simulink model "model_sim_CHBjt5"  (R2023b)
settings: Solver=FixedStepAuto  StartTime=0.0  StopTime=5  FixedStep=1e-6  RelTol=1e-3
InitFcn:
  | sysinit
StopFcn:
  | code_CHBJT5_stopfcn
values from neighbouring files (symbols this model uses):
  C = 0.0234    [sysinit.m]
  f = 50    [sysinit.m]
  f_switch = 250    [sysinit.m]
  fn = 50    [sysinit.m]
  L = 0.002    [sysinit.m]
  L_ori = 0.02    [sysinit.m]
  L_sec = 0.06    [sysinit.m]
  m = 0.95    [sysinit.m]
  P0 = 8e6    (= 8000000)    [sysinit.m]
  R = 1.5    [sysinit.m]
  Source_Amp = 10000    [sysinit.m]
  st = 1e-6    (= 1e-06)    [sysinit.m]
  Td = 15e-7    (= 1.5e-06)    [sysinit.m]
  Ts2 = 0.5e-3    (= 0.0005)    [sysinit.m]
  U_dcN = 2500    [sysinit.m]
  Ul_in = 1900    [sysinit.m]
undefined symbols (not defined in the file or in its folder): D1, Delta, magnitude
libraries: spsSeriesRLCBranchLib x63, spsDiodeLib x30, simulink x26, spsIGBTLib x24, spsMeanLib x20, spsCurrentMeasurementLib x10, spsThreePhaseVIMeasurementLib x7, spsOnDelayLib x6, spsUniversalBridgeLib x6, spsRMSLib x4, spsVoltageMeasurementLib x3, spsThreePhaseTransformerThreeWindingsLib x3
(part 1 of 2)
settings Model: SimulationMode=accelerator  Creator=Jhchen  LastModifiedBy=Jhchen
settings DataIOCC: ReturnWorkspaceOutputs=off
settings DebuggingCC: RTPrefix=warning

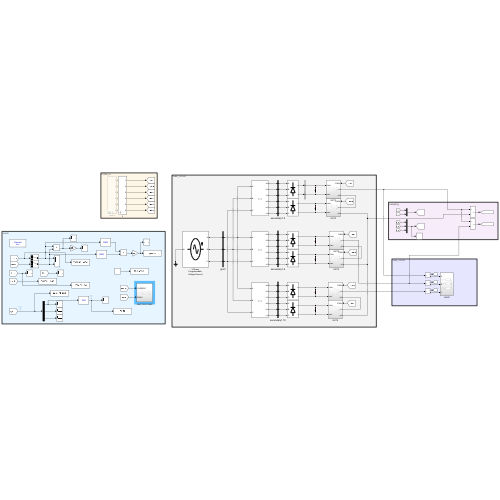
[thumbnail: Simulink's stored preview of the top-level diagram]
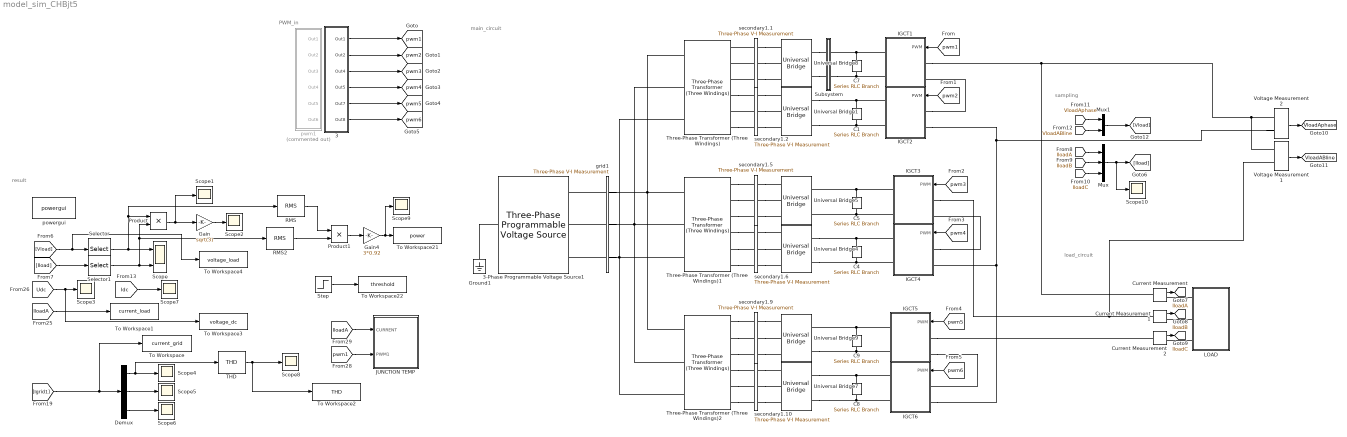
== system model_sim_CHBjt5 ==
  note: load_circuit
  note: main_circuit
  note: PWM_in
  note: result
  note: sampling
  3 : Subsystem  mask{m=m, f=f, f_car=f_switch, tt=1/4, ttd=Td}
      mask prompts: m "m_p"; f "f_module"; f_car "f_carrier"; tt "ts"; ttd "td"
      mask DialogControl ParameterGroupVar Prompt: 参数
  3-Phase Programmable Voltage Source1 : spsThreePhaseProgrammableVoltageSourceLib/Three-Phase Programmable Voltage Source  PositiveSequence=[10000 0 50]  VariationEntity=None  VariationType=Step  VariationTypeAlt=Step  VariationStep=0.5  VariationRate=10  VariationMagnitude=0.3  VariationFrequency=2  VariationTiming=[0.05 1]  VariationPhaseA=off  Amplitudes=[1 0.8 1.2 1.0]  TimeValues=[0 0.1 0.15 0.2]  HarmonicGeneration=off  HarmonicA=[5 0.08 -45 2]  HarmonicB=[2 0 0 2]  Timing="[0.1  1]"  BusType=swing  Pref=0  Qref=0  Qmin=-inf  Qmax=inf
  C{1,4..5,7..9} (6 alike) : spsSeriesRLCBranchLib/Series RLC Branch  LConnTagsString=__new0  RConnTagsString=__new0  BranchType=C  Resistance=0.0001  Inductance=1.0  SetiL0=off  InitialCurrent=0  Capacitance=C  Setx0=on  InitialVoltage=2500  Measurements=None
  Current Measurement : spsCurrentMeasurementLib/Current Measurement  PhasorSimulation=off  OutputType=Complex  PSBequivalent=0
  Current Measurement1 : spsCurrentMeasurementLib/Current Measurement  PhasorSimulation=off  OutputType=Complex  PSBequivalent=0
  Current Measurement2 : spsCurrentMeasurementLib/Current Measurement  PhasorSimulation=off  OutputType=Complex  PSBequivalent=0
  Demux : Demux  Outputs=3
  Gain : Gain  Gain=sqrt(3)
  Gain4 : Gain  Gain=3*0.92
  Ground1 : spsGroundLib/Ground  LConnTagsString=a
  IGCT1 : Subsystem
      settings: PortSchema="{\"entries\":[{\"content\":{\"sides\":[{\"content\":{\"connectorIds\":[\"LConn1\",\"LConn2\"]},\"type\":\"ConnectorPlacement.EquallySpacedRectSide\",\"uuid\":\"3b5227fd-32cc-4097-9a6a-2909540651e9\"},{\"content\":{\"connectorIds\":[\"In1\",\"RConn1\",\"RConn2\"],\"side\":\"RIGHT\"},\"type\":\"ConnectorPlacement.EquallySpacedRectSide\",\"uuid\":\"b0068562-9d9a-456b-acd2-db870c5bcace\"},{\"content\":{\"side\":\"TOP\"},\"type\":\"ConnectorPlacement.EquallySpacedRectSide\",\"uuid\":\"bbecbe08-a8e7-4703-9f6f-443f87d924da\"}]},\"type\":\"ConnectorPlacement.EquallySpacedConnector\",\"uuid\":\"6ec83c7b-e3bb-4502-bc8f-4da9ff103a20\"}],\"packageUris\":[\"http://schema.mathworks.com/mf0/Connector/R2020b\"],\"version\":\"1.0\"}"
  IGCT2 : Subsystem
      settings: PortSchema="{\"entries\":[{\"content\":{\"sides\":[{\"content\":{\"connectorIds\":[\"LConn1\",\"LConn2\"]},\"type\":\"ConnectorPlacement.EquallySpacedRectSide\",\"uuid\":\"3b5227fd-32cc-4097-9a6a-2909540651e9\"},{\"content\":{\"connectorIds\":[\"In1\",\"RConn1\",\"RConn2\"],\"side\":\"RIGHT\"},\"type\":\"ConnectorPlacement.EquallySpacedRectSide\",\"uuid\":\"b0068562-9d9a-456b-acd2-db870c5bcace\"},{\"content\":{\"side\":\"TOP\"},\"type\":\"ConnectorPlacement.EquallySpacedRectSide\",\"uuid\":\"bbecbe08-a8e7-4703-9f6f-443f87d924da\"}]},\"type\":\"ConnectorPlacement.EquallySpacedConnector\",\"uuid\":\"6ec83c7b-e3bb-4502-bc8f-4da9ff103a20\"}],\"packageUris\":[\"http://schema.mathworks.com/mf0/Connector/R2020b\"],\"version\":\"1.0\"}"
  IGCT3 : Subsystem
      settings: PortSchema="{\"entries\":[{\"content\":{\"sides\":[{\"content\":{\"connectorIds\":[\"LConn1\",\"LConn2\"]},\"type\":\"ConnectorPlacement.EquallySpacedRectSide\",\"uuid\":\"3b5227fd-32cc-4097-9a6a-2909540651e9\"},{\"content\":{\"connectorIds\":[\"In1\",\"RConn1\",\"RConn2\"],\"side\":\"RIGHT\"},\"type\":\"ConnectorPlacement.EquallySpacedRectSide\",\"uuid\":\"b0068562-9d9a-456b-acd2-db870c5bcace\"},{\"content\":{\"side\":\"TOP\"},\"type\":\"ConnectorPlacement.EquallySpacedRectSide\",\"uuid\":\"bbecbe08-a8e7-4703-9f6f-443f87d924da\"}]},\"type\":\"ConnectorPlacement.EquallySpacedConnector\",\"uuid\":\"6ec83c7b-e3bb-4502-bc8f-4da9ff103a20\"}],\"packageUris\":[\"http://schema.mathworks.com/mf0/Connector/R2020b\"],\"version\":\"1.0\"}"
  IGCT4 : Subsystem
      settings: PortSchema="{\"entries\":[{\"content\":{\"sides\":[{\"content\":{\"connectorIds\":[\"LConn1\",\"LConn2\"]},\"type\":\"ConnectorPlacement.EquallySpacedRectSide\",\"uuid\":\"3b5227fd-32cc-4097-9a6a-2909540651e9\"},{\"content\":{\"connectorIds\":[\"In1\",\"RConn1\",\"RConn2\"],\"side\":\"RIGHT\"},\"type\":\"ConnectorPlacement.EquallySpacedRectSide\",\"uuid\":\"b0068562-9d9a-456b-acd2-db870c5bcace\"},{\"content\":{\"side\":\"TOP\"},\"type\":\"ConnectorPlacement.EquallySpacedRectSide\",\"uuid\":\"bbecbe08-a8e7-4703-9f6f-443f87d924da\"}]},\"type\":\"ConnectorPlacement.EquallySpacedConnector\",\"uuid\":\"6ec83c7b-e3bb-4502-bc8f-4da9ff103a20\"}],\"packageUris\":[\"http://schema.mathworks.com/mf0/Connector/R2020b\"],\"version\":\"1.0\"}"
  IGCT5 : Subsystem
      settings: PortSchema="{\"entries\":[{\"content\":{\"sides\":[{\"content\":{\"connectorIds\":[\"LConn1\",\"LConn2\"]},\"type\":\"ConnectorPlacement.EquallySpacedRectSide\",\"uuid\":\"3b5227fd-32cc-4097-9a6a-2909540651e9\"},{\"content\":{\"connectorIds\":[\"In1\",\"RConn1\",\"RConn2\"],\"side\":\"RIGHT\"},\"type\":\"ConnectorPlacement.EquallySpacedRectSide\",\"uuid\":\"b0068562-9d9a-456b-acd2-db870c5bcace\"},{\"content\":{\"side\":\"TOP\"},\"type\":\"ConnectorPlacement.EquallySpacedRectSide\",\"uuid\":\"bbecbe08-a8e7-4703-9f6f-443f87d924da\"}]},\"type\":\"ConnectorPlacement.EquallySpacedConnector\",\"uuid\":\"6ec83c7b-e3bb-4502-bc8f-4da9ff103a20\"}],\"packageUris\":[\"http://schema.mathworks.com/mf0/Connector/R2020b\"],\"version\":\"1.0\"}"
  IGCT6 : Subsystem
      settings: PortSchema="{\"entries\":[{\"content\":{\"sides\":[{\"content\":{\"connectorIds\":[\"LConn1\",\"LConn2\"]},\"type\":\"ConnectorPlacement.EquallySpacedRectSide\",\"uuid\":\"3b5227fd-32cc-4097-9a6a-2909540651e9\"},{\"content\":{\"connectorIds\":[\"In1\",\"RConn1\",\"RConn2\"],\"side\":\"RIGHT\"},\"type\":\"ConnectorPlacement.EquallySpacedRectSide\",\"uuid\":\"b0068562-9d9a-456b-acd2-db870c5bcace\"},{\"content\":{\"side\":\"TOP\"},\"type\":\"ConnectorPlacement.EquallySpacedRectSide\",\"uuid\":\"bbecbe08-a8e7-4703-9f6f-443f87d924da\"}]},\"type\":\"ConnectorPlacement.EquallySpacedConnector\",\"uuid\":\"6ec83c7b-e3bb-4502-bc8f-4da9ff103a20\"}],\"packageUris\":[\"http://schema.mathworks.com/mf0/Connector/R2020b\"],\"version\":\"1.0\"}"
  JUNCTION TEMP : Subsystem
  LOAD : Subsystem
  Mux : Mux  Inputs=3
  Mux1 : Mux  Inputs=2
  Product : Product
  Product1 : Product
  RMS : spsRMSLib/RMS  TrueRMS=on  Freq=f  RMSInit=0  Ts=0
  RMS2 : spsRMSLib/RMS  TrueRMS=on  Freq=f  RMSInit=0  Ts=0
  Scope : Scope  NumInputPorts=2
  Scope{1..10} (10 alike) : Scope
  Selector : Selector  InputPortWidth=2  IndexOptions=Index vector (dialog)  Indices=[1]  OutputSizes=1
  Selector1 : Selector  InputPortWidth=3  IndexOptions=Index vector (dialog)  Indices=[1]  OutputSizes=1
  Step : Step  Time=0  Before=140  After=140  SampleTime=0
  Subsystem : Subsystem
  THD : spsTHDLib/THD  Freq=f  Ts=0
  Three-Phase Transformer (Three Windings) : spsThreePhaseTransformerThreeWindingsLib/Three-Phase Transformer (Three Windings)  Winding1Connection=Y  Winding2Connection=Y  Winding3Connection=Delta (D1)  CoreType=Three single-phase transformers  SetSaturation=off  Hysteresis=off  DataFile='hysteresis'  SetInitialFlux=off  Measurements=None  UNITS=pu  NominalPower=[ P0, fn ]  Winding1=[Source_Amp 0.002 L_ori]  Winding2=[Ul_in 0.002 L_sec]  Winding3=[Ul_in 0.002 L_sec]  Rm=500  Lm=499.99  L0=0.5  Saturation=[0 0;0.0024 1.2;1 1.5199]  InitialFluxes=[0.8 -0.8 0.7]  BreakLoop=off  DiscreteSolver=Trapezoidal iterative  DataType=off  TransfoNumber=1
      settings: LibrarySourceBlock=|
      | sps_lib/Power Grid Elements/Three-Phase
      | Transformer
      | (Three Windings)
  Three-Phase Transformer (Three Windings)1 : spsThreePhaseTransformerThreeWindingsLib/Three-Phase Transformer (Three Windings)  Winding1Connection=Y  Winding2Connection=Y  Winding3Connection=Delta (D1)  CoreType=Three single-phase transformers  SetSaturation=off  Hysteresis=off  DataFile='hysteresis'  SetInitialFlux=off  Measurements=None  UNITS=pu  NominalPower=[ P0, fn ]  Winding1=[Source_Amp 0.002 L_ori]  Winding2=[Ul_in 0.002 L_sec]  Winding3=[Ul_in 0.002 L_sec]  Rm=500  Lm=499.99  L0=0.5  Saturation=[0 0;0.0024 1.2;1 1.5199]  InitialFluxes=[0.8 -0.8 0.7]  BreakLoop=off  DiscreteSolver=Trapezoidal iterative  DataType=off  TransfoNumber=1
      settings: LibrarySourceBlock=|
      | sps_lib/Power Grid Elements/Three-Phase
      | Transformer
      | (Three Windings)
  Three-Phase Transformer (Three Windings)2 : spsThreePhaseTransformerThreeWindingsLib/Three-Phase Transformer (Three Windings)  Winding1Connection=Y  Winding2Connection=Y  Winding3Connection=Delta (D1)  CoreType=Three single-phase transformers  SetSaturation=off  Hysteresis=off  DataFile='hysteresis'  SetInitialFlux=off  Measurements=None  UNITS=pu  NominalPower=[ P0, fn ]  Winding1=[Source_Amp 0.002 L_ori]  Winding2=[Ul_in 0.002 L_sec]  Winding3=[Ul_in 0.002 L_sec]  Rm=500  Lm=499.99  L0=0.5  Saturation=[0 0;0.0024 1.2;1 1.5199]  InitialFluxes=[0.8 -0.8 0.7]  BreakLoop=off  DiscreteSolver=Trapezoidal iterative  DataType=off  TransfoNumber=1
      settings: LibrarySourceBlock=|
      | sps_lib/Power Grid Elements/Three-Phase
      | Transformer
      | (Three Windings)
  To Workspace : ToWorkspace  VariableName=current_grid  SaveFormat=Structure With Time  SampleTime=-1
  To Workspace1 : ToWorkspace  VariableName=current_load  SaveFormat=Structure With Time  SampleTime=-1
  To Workspace2 : ToWorkspace  VariableName=THD  SaveFormat=Structure With Time  SampleTime=-1
  To Workspace21 : ToWorkspace  VariableName=power  SaveFormat=Structure With Time  SampleTime=-1
  To Workspace22 : ToWorkspace  VariableName=threshold  SaveFormat=Structure With Time  SampleTime=-1
  To Workspace3 : ToWorkspace  VariableName=voltage_dc  SaveFormat=Structure With Time  SampleTime=-1
  To Workspace4 : ToWorkspace  VariableName=voltage_load  SaveFormat=Structure With Time  SampleTime=-1
  Universal Bridge{1,4..5,7..9} (6 alike) : spsUniversalBridgeLib/Universal Bridge  Arms=3  SnubberResistance=1e5  SnubberCapacitance=inf  Device=Diodes  Ron=1e-3  Lon=0  ForwardVoltages="[  0  0  ]"  ForwardVoltage=0  GTOparameters=[ 10e-6 , 20e-6 ]  IGBTparameters=[ 1e-6 , 2e-6 ]  Measurements=None  Measurements_2=None  converterType=Rectifier
  Voltage Measurement1 : spsVoltageMeasurementLib/Voltage Measurement  PhasorSimulation=off  OutputType=Complex  PSBequivalent=0
  Voltage Measurement2 : spsVoltageMeasurementLib/Voltage Measurement  PhasorSimulation=off  OutputType=Complex  PSBequivalent=0
  grid1 : spsThreePhaseVIMeasurementLib/Three-Phase V-I Measurement  VoltageMeasurement=phase-to-ground  SetLabelV=on  LabelV=Vgrid1  Vpu=off  VpuLL=off  CurrentMeasurement=yes  SetLabelI=on  LabelI=Igrid1  Ipu=off  Pbase=1e3  Vbase=380  OutputType=Magnitude  PhasorSimulation=off  PSBequivalent=0
  powergui : spspowerguiLib/powergui  Priority=1  SimulationMode=Discrete  SampleTime=st  frequency=60  Iterations=50  frequencyindice=50  Pbase=100e6  ErrMax=1e-4  UnitsV=kV  UnitsW=MW  buscounter=0  FunctionMessages=off  echomessages=off  EnableUseOfTLC=off  CurrentSourceSwitches=off  DisableSnubberDevices=off  DisableRonSwitches=off  DisableVfSwitches=off  DisplayEquations=off  AutomaticDiscreteSolvers=off  SolverType=Tustin/Backward Euler (TBE)  Interpol=off  ExternalGateDelay=off  methode=off  Ts=100  x0status=blocks  SPID=on  SwTol=0  HookPort=off  NonlinearTolerance=1e-4  nMaxIteration=100  ContinueOnMaxIteration=off  RestoreLinks=warning  ResistiveCurrentMeasurement=off  Frange=[0:2:500]  Ylog=off  Xlog=on  ShowGrid=off  save=off  variable=ZData  structure=0  ZoomFFT=off  StartTime=0.0  cycles=1  DisplayStyle=1  fundamental=60  FreqAxis=off  MaxFrequency=1000  frequencyindicesteady=1  RmsSteady=1  display=off
  pwm1 : Subsystem  Commented=on  mask{m=0.95, f=50, f_carrier=250, sw1=TRIBLE_SINE, sw=PS4}
      mask prompts: m "m_p"; f "f_module"; sw1 "mod"; sw "pwm_out"
      mask TypeOptions sw1: SINE | TRIBLE_SINE | GDSINE1 | GDSINE2
      mask TypeOptions sw: PS4 | POD1 | PD2
  secondary1.1 : spsThreePhaseVIMeasurementLib/Three-Phase V-I Measurement  VoltageMeasurement=phase-to-phase  SetLabelV=on  LabelV=Vsecondary_a1  Vpu=off  VpuLL=off  CurrentMeasurement=yes  SetLabelI=on  LabelI=Isecondary_a1  Ipu=off  Pbase=1e3  Vbase=380  OutputType=Magnitude  PhasorSimulation=off  PSBequivalent=0
  secondary1.10 : spsThreePhaseVIMeasurementLib/Three-Phase V-I Measurement  VoltageMeasurement=phase-to-phase  SetLabelV=on  LabelV=Vsecondary_c2  Vpu=off  VpuLL=off  CurrentMeasurement=yes  SetLabelI=on  LabelI=Isecondary_c2  Ipu=off  Pbase=1e3  Vbase=380  OutputType=Magnitude  PhasorSimulation=off  PSBequivalent=0
  secondary1.2 : spsThreePhaseVIMeasurementLib/Three-Phase V-I Measurement  VoltageMeasurement=phase-to-phase  SetLabelV=on  LabelV=Vsecondary_a2  Vpu=off  VpuLL=off  CurrentMeasurement=yes  SetLabelI=on  LabelI=Isecondary_a2  Ipu=off  Pbase=1e3  Vbase=380  OutputType=Magnitude  PhasorSimulation=off  PSBequivalent=0
  secondary1.5 : spsThreePhaseVIMeasurementLib/Three-Phase V-I Measurement  VoltageMeasurement=phase-to-phase  SetLabelV=on  LabelV=Vsecondary_b1  Vpu=off  VpuLL=off  CurrentMeasurement=yes  SetLabelI=on  LabelI=Isecondary_b1  Ipu=off  Pbase=1e3  Vbase=380  OutputType=Magnitude  PhasorSimulation=off  PSBequivalent=0
  secondary1.6 : spsThreePhaseVIMeasurementLib/Three-Phase V-I Measurement  VoltageMeasurement=phase-to-phase  SetLabelV=on  LabelV=Vsecondary_b2  Vpu=off  VpuLL=off  CurrentMeasurement=yes  SetLabelI=on  LabelI=Isecondary_b2  Ipu=off  Pbase=1e3  Vbase=380  OutputType=Magnitude  PhasorSimulation=off  PSBequivalent=0
  secondary1.9 : spsThreePhaseVIMeasurementLib/Three-Phase V-I Measurement  VoltageMeasurement=phase-to-phase  SetLabelV=on  LabelV=Vsecondary_c1  Vpu=off  VpuLL=off  CurrentMeasurement=yes  SetLabelI=on  LabelI=Isecondary_c1  Ipu=off  Pbase=1e3  Vbase=380  OutputType=Magnitude  PhasorSimulation=off  PSBequivalent=0
  tag scope: IloadA=global, IloadB=global, IloadC=global, VloadABline=global, VloadAphase=global, pwm1=global, pwm2=global, pwm3=global, pwm4=global, pwm5=global, pwm6=global
  wires:
  [pwm1] -> IGCT1/1(PWM)
  [pwm2] -> IGCT2/1(PWM)
  [pwm3] -> IGCT3/1(PWM)
  [pwm4] -> IGCT4/1(PWM)
  [pwm5] -> IGCT5/1(PWM)
  [pwm6] -> IGCT6/1(PWM)
  [Vload] -> To Workspace4/1, Selector/1
  Selector/1 -> Product/1, RMS/1, Scope/1
  [Iload] -> Selector1/1
  Selector1/1 -> Product/2, RMS2/1, Scope/2
  Current Measurement/1 -> [IloadA]
  Current Measurement1/1 -> [IloadB]
  Current Measurement2/1 -> [IloadC]
  [IloadC] -> Mux/3
  [IloadB] -> Mux/2
  [IloadA] -> Mux/1
  Mux/1 -> Scope10/1, [Iload]
  Voltage Measurement2/1 -> [VloadAphase]
  Voltage Measurement1/1 -> [VloadABline]
  [VloadAphase] -> Mux1/1
  [VloadABline] -> Mux1/2
  Mux1/1 -> [Vload]
  Product/1 -> Scope1/1, Gain/1
  Gain/1 -> Scope2/1
  [IloadA] -> To Workspace1/1
  [Udc] -> To Workspace3/1, Scope3/1
  3/1(Out1) -> [pwm1]
  3/2(Out2) -> [pwm2]
  3/3(Out4) -> [pwm3]
  3/4(Out5) -> [pwm4]
  3/5(Out7) -> [pwm5]
  3/6(Out8) -> [pwm6]
  [Igrid1] -> Demux/1, To Workspace/1
  Demux/1 -> THD/1, Scope4/1
  Demux/2 -> Scope5/1
  Demux/3 -> Scope6/1
  [Idc] -> Scope7/1
  THD/1 -> To Workspace2/1, Scope8/1
  RMS/1 -> Product1/1
  RMS2/1 -> Product1/2
  Product1/1 -> Gain4/1
  Gain4/1 -> Scope9/1, To Workspace21/1
  Step/1 -> To Workspace22/1
  [IloadA] -> JUNCTION TEMP/1(CURRENT)
  [pwm1] -> JUNCTION TEMP/2(PWM1)
  connections:
  grid1/LConn3 -- 3-Phase Programmable Voltage Source1/RConn3
  grid1/LConn2 -- 3-Phase Programmable Voltage Source1/RConn2
  grid1/RConn3 -- Three-Phase Transformer (Three Windings)2/LConn3 -- Three-Phase Transformer (Three Windings)1/LConn3 -- Three-Phase Transformer (Three Windings)/LConn3
  grid1/RConn2 -- Three-Phase Transformer (Three Windings)2/LConn2 -- Three-Phase Transformer (Three Windings)1/LConn2 -- Three-Phase Transformer (Three Windings)/LConn2
  secondary1.1/RConn2 -- Universal Bridge8/LConn2
  Three-Phase Transformer (Three Windings)/RConn6 -- secondary1.2/LConn3
  secondary1.2/LConn2 -- Three-Phase Transformer (Three Windings)/RConn5
  Three-Phase Transformer (Three Windings)/RConn4 -- secondary1.2/LConn1
  secondary1.1/LConn3 -- Three-Phase Transformer (Three Windings)/RConn3
  secondary1.1/LConn2 -- Three-Phase Transformer (Three Windings)/RConn2
  secondary1.1/RConn3 -- Universal Bridge8/LConn3
  secondary1.2/RConn1 -- Universal Bridge1/LConn1
  secondary1.2/RConn2 -- Universal Bridge1/LConn2
  secondary1.2/RConn3 -- Universal Bridge1/LConn3
  secondary1.1/RConn1 -- Universal Bridge8/LConn1
  secondary1.1/LConn1 -- Three-Phase Transformer (Three Windings)/RConn1
  Universal Bridge1/RConn2 -- IGCT2/LConn2 -- C1/RConn1
  Universal Bridge1/RConn1 -- IGCT2/LConn1 -- C1/LConn1
  Universal Bridge8/RConn1 -- Subsystem/LConn1
  Universal Bridge8/RConn2 -- Subsystem/LConn2
  Subsystem/RConn2 -- IGCT1/LConn2 -- C7/RConn1
  C7/LConn1 -- IGCT1/LConn1 -- Subsystem/RConn1
  IGCT2/RConn1 -- IGCT1/RConn2
  Universal Bridge4/RConn2 -- IGCT4/LConn2 -- C4/RConn1
  Universal Bridge4/RConn1 -- IGCT4/LConn1 -- C4/LConn1
  secondary1.5/RConn2 -- Universal Bridge5/LConn2
  Three-Phase Transformer (Three Windings)1/RConn1 -- secondary1.5/LConn1
  Three-Phase Transformer (Three Windings)1/RConn2 -- secondary1.5/LConn2
  Three-Phase Transformer (Three Windings)1/RConn5 -- secondary1.6/LConn2
  Three-Phase Transformer (Three Windings)1/RConn3 -- secondary1.5/LConn3
  Three-Phase Transformer (Three Windings)1/RConn6 -- secondary1.6/LConn3
  secondary1.6/RConn1 -- Universal Bridge4/LConn1
  secondary1.6/RConn2 -- Universal Bridge4/LConn2
  secondary1.6/RConn3 -- Universal Bridge4/LConn3
  C5/LConn1 -- Universal Bridge5/RConn1 -- IGCT3/LConn1
  secondary1.5/RConn1 -- Universal Bridge5/LConn1
  C5/RConn1 -- Universal Bridge5/RConn2 -- IGCT3/LConn2
  secondary1.5/RConn3 -- Universal Bridge5/LConn3
  Three-Phase Transformer (Three Windings)1/RConn4 -- secondary1.6/LConn1
  grid1/RConn1 -- Three-Phase Transformer (Three Windings)2/LConn1 -- Three-Phase Transformer (Three Windings)1/LConn1 -- Three-Phase Transformer (Three Windings)/LConn1
  grid1/LConn1 -- 3-Phase Programmable Voltage Source1/RConn1
  LOAD/LConn2 -- Current Measurement1/RConn1
  Current Measurement/RConn1 -- LOAD/LConn1
  Current Measurement2/RConn1 -- LOAD/LConn3
  Universal Bridge7/RConn2 -- IGCT6/LConn2 -- C8/RConn1
  Universal Bridge7/RConn1 -- IGCT6/LConn1 -- C8/LConn1
  C9/RConn1 -- IGCT5/LConn2 -- Universal Bridge9/RConn2
  C9/LConn1 -- IGCT5/LConn1 -- Universal Bridge9/RConn1
  secondary1.9/RConn2 -- Universal Bridge9/LConn2
  Three-Phase Transformer (Three Windings)2/RConn1 -- secondary1.9/LConn1
  Three-Phase Transformer (Three Windings)2/RConn6 -- secondary1.10/LConn3
  Three-Phase Transformer (Three Windings)2/RConn2 -- secondary1.9/LConn2
  Three-Phase Transformer (Three Windings)2/RConn5 -- secondary1.10/LConn2
  Three-Phase Transformer (Three Windings)2/RConn3 -- secondary1.9/LConn3
  secondary1.9/RConn3 -- Universal Bridge9/LConn3
  secondary1.10/RConn2 -- Universal Bridge7/LConn2
  secondary1.10/RConn3 -- Universal Bridge7/LConn3
  Three-Phase Transformer (Three Windings)2/RConn4 -- secondary1.10/LConn1
  secondary1.10/RConn1 -- Universal Bridge7/LConn1
  secondary1.9/RConn1 -- Universal Bridge9/LConn1
  IGCT4/RConn1 -- IGCT3/RConn2
  Current Measurement/LConn1 -- Voltage Measurement1/LConn1 -- Voltage Measurement2/LConn1 -- IGCT1/RConn1
  Voltage Measurement1/LConn2 -- IGCT3/RConn1 -- Current Measurement1/LConn1
  IGCT5/RConn2 -- IGCT6/RConn1
  IGCT5/RConn1 -- Current Measurement2/LConn1
  IGCT2/RConn2 -- Voltage Measurement2/LConn2 -- IGCT6/RConn2 -- IGCT4/RConn2
  Ground1/LConn1 -- 3-Phase Programmable Voltage Source1/LConn1

== system model_sim_CHBjt5/3 ==
  -2/3*pi : Subsystem
  0 : Subsystem
  2/3*pi : Subsystem
  Sine Wave : Sin  Amplitude=m*1000  Frequency=f*2*pi  Phase=2/3*pi  SampleTime=0
  Sine Wave1 : Sin  Amplitude=m*1000  Frequency=f*2*pi  SampleTime=0
  Sine Wave2 : Sin  Amplitude=m*1000  Frequency=f*2*pi  Phase=-2/3*pi  SampleTime=0
  Subsystem : Subsystem
  Out1 : Outport
  Out2 : Outport  Port=2
  Out4 : Outport  Port=3
  Out5 : Outport  Port=4
  Out7 : Outport  Port=5
  Out8 : Outport  Port=6
  wires:
  Subsystem/3(Out3) -> -2/3*pi/1(In1)
  Subsystem/2(Out2) -> 0/1(In1)
  Subsystem/1(Out1) -> 2/3*pi/1(In1)
  Sine Wave2/1 -> Subsystem/3(In3)
  Sine Wave1/1 -> Subsystem/2(In2)
  Sine Wave/1 -> Subsystem/1(In1)
  -2/3*pi/1(Out1) -> Out7/1
  0/1(Out1) -> Out4/1
  -2/3*pi/2(Out2) -> Out8/1
  2/3*pi/1(Out1) -> Out1/1
  2/3*pi/2(Out2) -> Out2/1
  0/2(Out2) -> Out5/1

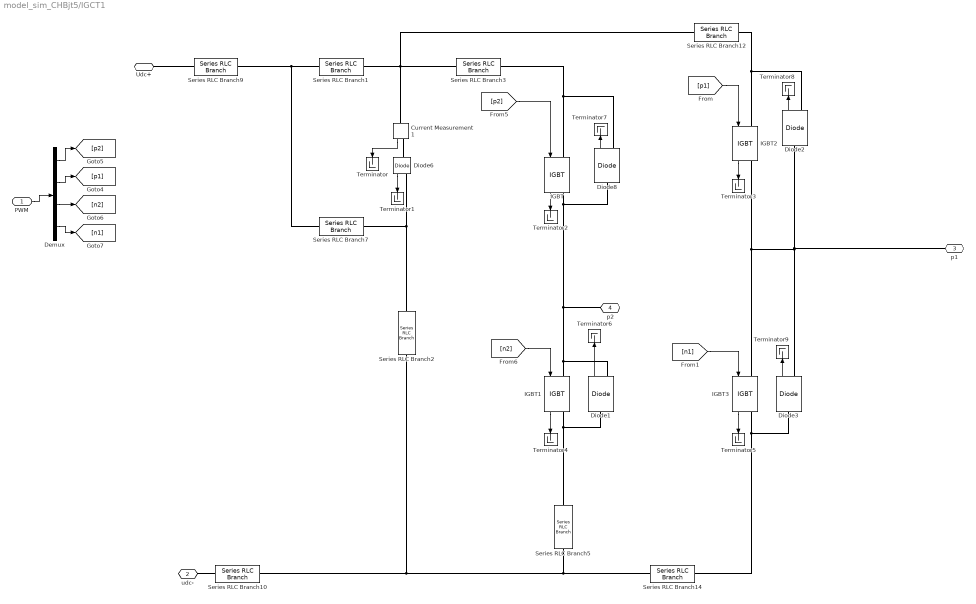
== system model_sim_CHBjt5/IGCT1 ==
  PWM : Inport
  Current Measurement1 : spsCurrentMeasurementLib/Current Measurement  PhasorSimulation=off  OutputType=Complex  PSBequivalent=0
  Demux : Demux
  Diode{1..3,6,8} (5 alike) : spsDiodeLib/Diode  Ron=rto  Lon=0  Vf=vto  IC=0  UseSnubber=off  Rs=500  Cs=250e-9  Measurements=on
  IGBT{,1..3} (4 alike) : spsIGBTLib/IGBT  Ron=rt  Lon=0  Vf=vt  Tf=1e-6  Tt=2e-6  IC=0  Rs=1e5  Cs=inf  Measurements=on
  Series RLC Branch1 : spsSeriesRLCBranchLib/Series RLC Branch  LConnTagsString=__new0  RConnTagsString=__new0  BranchType=RL  Resistance=1e-5  Inductance=3.0E-6  SetiL0=off  InitialCurrent=0  Capacitance=1e-6  Setx0=off  InitialVoltage=0  Measurements=None
  Series RLC Branch10 : spsSeriesRLCBranchLib/Series RLC Branch  LConnTagsString=__new0  RConnTagsString=__new0  BranchType=L  Resistance=1  Inductance=0.4e-6  SetiL0=off  InitialCurrent=0  Capacitance=1e-6  Setx0=off  InitialVoltage=0  Measurements=None
  Series RLC Branch12 : spsSeriesRLCBranchLib/Series RLC Branch  LConnTagsString=__new0  RConnTagsString=__new0  BranchType=RL  Resistance=1e-5  Inductance=1E-9  SetiL0=off  InitialCurrent=0  Capacitance=1e-6  Setx0=off  InitialVoltage=0  Measurements=None
  Series RLC Branch14 : spsSeriesRLCBranchLib/Series RLC Branch  LConnTagsString=__new0  RConnTagsString=__new0  BranchType=L  Resistance=1  Inductance=1E-7  SetiL0=off  InitialCurrent=0  Capacitance=1e-6  Setx0=off  InitialVoltage=0  Measurements=None
  Series RLC Branch2 : spsSeriesRLCBranchLib/Series RLC Branch  LConnTagsString=__new0  RConnTagsString=__new0  BranchType=RC  Resistance=1e-5  Inductance=20e-6  SetiL0=off  InitialCurrent=0  Capacitance=17e-6  Setx0=off  InitialVoltage=0  Measurements=None
  Series RLC Branch3 : spsSeriesRLCBranchLib/Series RLC Branch  LConnTagsString=__new0  RConnTagsString=__new0  BranchType=RL  Resistance=1e-5  Inductance=1E-9  SetiL0=off  InitialCurrent=0  Capacitance=1e-6  Setx0=off  InitialVoltage=0  Measurements=None
  Series RLC Branch5 : spsSeriesRLCBranchLib/Series RLC Branch  LConnTagsString=__new0  RConnTagsString=__new0  BranchType=L  Resistance=1  Inductance=1E-7  SetiL0=off  InitialCurrent=0  Capacitance=1e-6  Setx0=off  InitialVoltage=0  Measurements=None
  Series RLC Branch7 : spsSeriesRLCBranchLib/Series RLC Branch  LConnTagsString=__new0  RConnTagsString=__new0  BranchType=RL  Resistance=0.6  Inductance=1e-6  SetiL0=off  InitialCurrent=0  Capacitance=1e-6  Setx0=off  InitialVoltage=0  Measurements=None
  Series RLC Branch9 : spsSeriesRLCBranchLib/Series RLC Branch  LConnTagsString=__new0  RConnTagsString=__new0  BranchType=L  Resistance=1  Inductance=0.4e-6  SetiL0=off  InitialCurrent=0  Capacitance=1e-6  Setx0=off  InitialVoltage=0  Measurements=None
  Terminator{,1..9} (10 alike) : Terminator
  Udc+ : PMIOPort  Side=Left
  udc- : PMIOPort  Port=2  Side=Left
  p1 : PMIOPort  Port=3  Side=Right
  p2 : PMIOPort  Port=4  Side=Right
  wires:
  Diode3/1 -> Terminator9/1
  IGBT3/1 -> Terminator5/1
  [n1] -> IGBT3/1
  IGBT1/1 -> Terminator4/1
  IGBT2/1 -> Terminator3/1
  IGBT/1 -> Terminator2/1
  [n2] -> IGBT1/1
  [p1] -> IGBT2/1
  Current Measurement1/1 -> Terminator/1
  Diode2/1 -> Terminator8/1
  [p2] -> IGBT/1
  Diode8/1 -> Terminator7/1
  Diode1/1 -> Terminator6/1
  Diode6/1 -> Terminator1/1
  Demux/3 -> [n2]
  PWM/1 -> Demux/1
  Demux/1 -> [p2]
  Demux/2 -> [p1]
  Demux/4 -> [n1]
  connections:
  Series RLC Branch10/LConn1 -- udc-/RConn1
  Series RLC Branch9/LConn1 -- Udc+/RConn1
  Diode6/RConn1 -- Series RLC Branch7/RConn1 -- Series RLC Branch2/LConn1
  Current Measurement1/LConn1 -- Series RLC Branch1/RConn1 -- Series RLC Branch3/LConn1 -- Series RLC Branch12/LConn1
  Diode3/LConn1 -- IGBT3/RConn1 -- Series RLC Branch14/RConn1
  Series RLC Branch3/RConn1 -- IGBT/LConn1 -- Diode8/RConn1
  Diode1/LConn1 -- Series RLC Branch5/RConn1 -- IGBT1/RConn1
  Current Measurement1/RConn1 -- Diode6/LConn1
  Diode2/RConn1 -- Series RLC Branch12/RConn1 -- IGBT2/LConn1
  p1/RConn1 -- Diode2/LConn1 -- Diode3/RConn1 -- IGBT3/LConn1 -- IGBT2/RConn1
  Series RLC Branch5/LConn1 -- Series RLC Branch14/LConn1 -- Series RLC Branch10/RConn1 -- Series RLC Branch2/RConn1
  Series RLC Branch1/LConn1 -- Series RLC Branch7/LConn1 -- Series RLC Branch9/RConn1
  p2/RConn1 -- IGBT1/LConn1 -- Diode1/RConn1 -- Diode8/LConn1 -- IGBT/RConn1

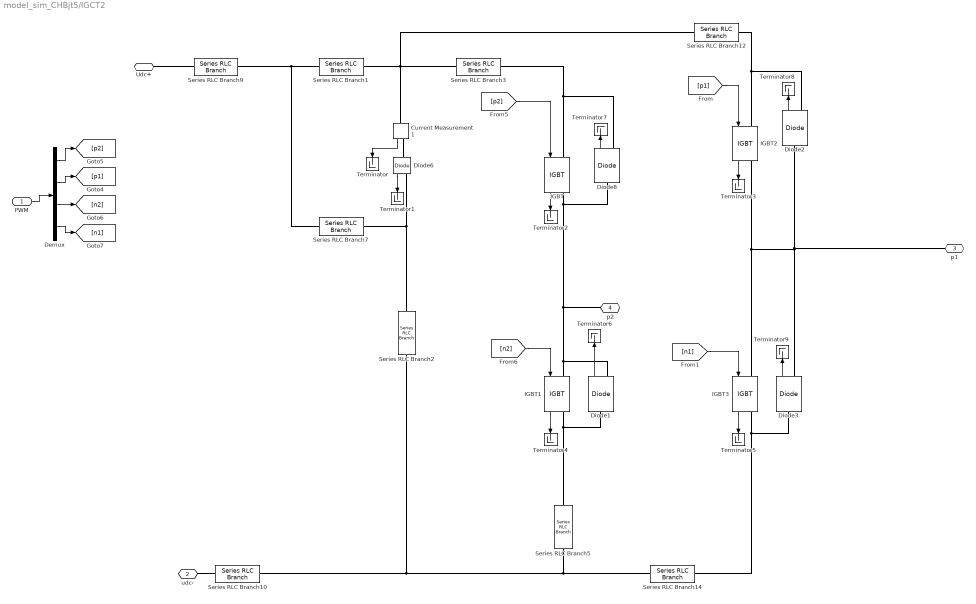
== system model_sim_CHBjt5/IGCT2 ==
  PWM : Inport
  Current Measurement1 : spsCurrentMeasurementLib/Current Measurement  PhasorSimulation=off  OutputType=Complex  PSBequivalent=0
  Demux : Demux
  Diode{1..3,6,8} (5 alike) : spsDiodeLib/Diode  Ron=rto  Lon=0  Vf=vto  IC=0  UseSnubber=off  Rs=500  Cs=250e-9  Measurements=on
  IGBT{,1..3} (4 alike) : spsIGBTLib/IGBT  Ron=rt  Lon=0  Vf=vt  Tf=1e-6  Tt=2e-6  IC=0  Rs=1e5  Cs=inf  Measurements=on
  Series RLC Branch1 : spsSeriesRLCBranchLib/Series RLC Branch  LConnTagsString=__new0  RConnTagsString=__new0  BranchType=RL  Resistance=1e-5  Inductance=3.0E-6  SetiL0=off  InitialCurrent=0  Capacitance=1e-6  Setx0=off  InitialVoltage=0  Measurements=None
  Series RLC Branch10 : spsSeriesRLCBranchLib/Series RLC Branch  LConnTagsString=__new0  RConnTagsString=__new0  BranchType=L  Resistance=1  Inductance=0.4e-6  SetiL0=off  InitialCurrent=0  Capacitance=1e-6  Setx0=off  InitialVoltage=0  Measurements=None
  Series RLC Branch12 : spsSeriesRLCBranchLib/Series RLC Branch  LConnTagsString=__new0  RConnTagsString=__new0  BranchType=RL  Resistance=1e-5  Inductance=1E-9  SetiL0=off  InitialCurrent=0  Capacitance=1e-6  Setx0=off  InitialVoltage=0  Measurements=None
  Series RLC Branch14 : spsSeriesRLCBranchLib/Series RLC Branch  LConnTagsString=__new0  RConnTagsString=__new0  BranchType=L  Resistance=1  Inductance=1E-7  SetiL0=off  InitialCurrent=0  Capacitance=1e-6  Setx0=off  InitialVoltage=0  Measurements=None
  Series RLC Branch2 : spsSeriesRLCBranchLib/Series RLC Branch  LConnTagsString=__new0  RConnTagsString=__new0  BranchType=RC  Resistance=1e-5  Inductance=20e-6  SetiL0=off  InitialCurrent=0  Capacitance=17e-6  Setx0=off  InitialVoltage=0  Measurements=None
  Series RLC Branch3 : spsSeriesRLCBranchLib/Series RLC Branch  LConnTagsString=__new0  RConnTagsString=__new0  BranchType=RL  Resistance=1e-5  Inductance=1E-9  SetiL0=off  InitialCurrent=0  Capacitance=1e-6  Setx0=off  InitialVoltage=0  Measurements=None
  Series RLC Branch5 : spsSeriesRLCBranchLib/Series RLC Branch  LConnTagsString=__new0  RConnTagsString=__new0  BranchType=L  Resistance=1  Inductance=1E-7  SetiL0=off  InitialCurrent=0  Capacitance=1e-6  Setx0=off  InitialVoltage=0  Measurements=None
  Series RLC Branch7 : spsSeriesRLCBranchLib/Series RLC Branch  LConnTagsString=__new0  RConnTagsString=__new0  BranchType=RL  Resistance=0.6  Inductance=1e-6  SetiL0=off  InitialCurrent=0  Capacitance=1e-6  Setx0=off  InitialVoltage=0  Measurements=None
  Series RLC Branch9 : spsSeriesRLCBranchLib/Series RLC Branch  LConnTagsString=__new0  RConnTagsString=__new0  BranchType=L  Resistance=1  Inductance=0.4e-6  SetiL0=off  InitialCurrent=0  Capacitance=1e-6  Setx0=off  InitialVoltage=0  Measurements=None
  Terminator{,1..9} (10 alike) : Terminator
  Udc+ : PMIOPort  Side=Left
  udc- : PMIOPort  Port=2  Side=Left
  p1 : PMIOPort  Port=3  Side=Right
  p2 : PMIOPort  Port=4  Side=Right
  wires:
  Diode3/1 -> Terminator9/1
  IGBT3/1 -> Terminator5/1
  [n1] -> IGBT3/1
  IGBT1/1 -> Terminator4/1
  IGBT2/1 -> Terminator3/1
  IGBT/1 -> Terminator2/1
  [n2] -> IGBT1/1
  [p1] -> IGBT2/1
  Current Measurement1/1 -> Terminator/1
  Diode2/1 -> Terminator8/1
  [p2] -> IGBT/1
  Diode8/1 -> Terminator7/1
  Diode1/1 -> Terminator6/1
  Diode6/1 -> Terminator1/1
  Demux/3 -> [n2]
  PWM/1 -> Demux/1
  Demux/1 -> [p2]
  Demux/2 -> [p1]
  Demux/4 -> [n1]
  connections:
  Series RLC Branch10/LConn1 -- udc-/RConn1
  Series RLC Branch9/LConn1 -- Udc+/RConn1
  Diode6/RConn1 -- Series RLC Branch7/RConn1 -- Series RLC Branch2/LConn1
  Current Measurement1/LConn1 -- Series RLC Branch1/RConn1 -- Series RLC Branch3/LConn1 -- Series RLC Branch12/LConn1
  Diode3/LConn1 -- IGBT3/RConn1 -- Series RLC Branch14/RConn1
  Series RLC Branch3/RConn1 -- IGBT/LConn1 -- Diode8/RConn1
  Diode1/LConn1 -- Series RLC Branch5/RConn1 -- IGBT1/RConn1
  Current Measurement1/RConn1 -- Diode6/LConn1
  Diode2/RConn1 -- Series RLC Branch12/RConn1 -- IGBT2/LConn1
  p1/RConn1 -- Diode2/LConn1 -- Diode3/RConn1 -- IGBT3/LConn1 -- IGBT2/RConn1
  Series RLC Branch5/LConn1 -- Series RLC Branch14/LConn1 -- Series RLC Branch10/RConn1 -- Series RLC Branch2/RConn1
  Series RLC Branch1/LConn1 -- Series RLC Branch7/LConn1 -- Series RLC Branch9/RConn1
  p2/RConn1 -- IGBT1/LConn1 -- Diode1/RConn1 -- Diode8/LConn1 -- IGBT/RConn1

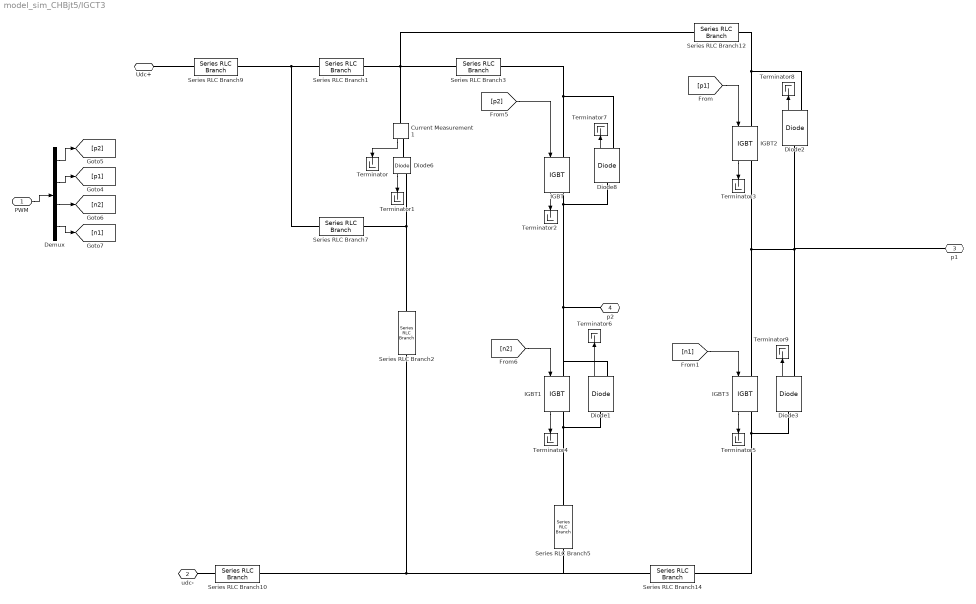
== system model_sim_CHBjt5/IGCT3 ==
  PWM : Inport
  Current Measurement1 : spsCurrentMeasurementLib/Current Measurement  PhasorSimulation=off  OutputType=Complex  PSBequivalent=0
  Demux : Demux
  Diode{1..3,6,8} (5 alike) : spsDiodeLib/Diode  Ron=rto  Lon=0  Vf=vto  IC=0  UseSnubber=off  Rs=500  Cs=250e-9  Measurements=on
  IGBT{,1..3} (4 alike) : spsIGBTLib/IGBT  Ron=rt  Lon=0  Vf=vt  Tf=1e-6  Tt=2e-6  IC=0  Rs=1e5  Cs=inf  Measurements=on
  Series RLC Branch1 : spsSeriesRLCBranchLib/Series RLC Branch  LConnTagsString=__new0  RConnTagsString=__new0  BranchType=RL  Resistance=1e-5  Inductance=3.0E-6  SetiL0=off  InitialCurrent=0  Capacitance=1e-6  Setx0=off  InitialVoltage=0  Measurements=None
  Series RLC Branch10 : spsSeriesRLCBranchLib/Series RLC Branch  LConnTagsString=__new0  RConnTagsString=__new0  BranchType=L  Resistance=1  Inductance=0.4e-6  SetiL0=off  InitialCurrent=0  Capacitance=1e-6  Setx0=off  InitialVoltage=0  Measurements=None
  Series RLC Branch12 : spsSeriesRLCBranchLib/Series RLC Branch  LConnTagsString=__new0  RConnTagsString=__new0  BranchType=RL  Resistance=1e-5  Inductance=1E-9  SetiL0=off  InitialCurrent=0  Capacitance=1e-6  Setx0=off  InitialVoltage=0  Measurements=None
  Series RLC Branch14 : spsSeriesRLCBranchLib/Series RLC Branch  LConnTagsString=__new0  RConnTagsString=__new0  BranchType=L  Resistance=1  Inductance=1E-7  SetiL0=off  InitialCurrent=0  Capacitance=1e-6  Setx0=off  InitialVoltage=0  Measurements=None
  Series RLC Branch2 : spsSeriesRLCBranchLib/Series RLC Branch  LConnTagsString=__new0  RConnTagsString=__new0  BranchType=RC  Resistance=1e-5  Inductance=20e-6  SetiL0=off  InitialCurrent=0  Capacitance=17e-6  Setx0=off  InitialVoltage=0  Measurements=None
  Series RLC Branch3 : spsSeriesRLCBranchLib/Series RLC Branch  LConnTagsString=__new0  RConnTagsString=__new0  BranchType=RL  Resistance=1e-5  Inductance=1E-9  SetiL0=off  InitialCurrent=0  Capacitance=1e-6  Setx0=off  InitialVoltage=0  Measurements=None
  Series RLC Branch5 : spsSeriesRLCBranchLib/Series RLC Branch  LConnTagsString=__new0  RConnTagsString=__new0  BranchType=L  Resistance=1  Inductance=1E-7  SetiL0=off  InitialCurrent=0  Capacitance=1e-6  Setx0=off  InitialVoltage=0  Measurements=None
  Series RLC Branch7 : spsSeriesRLCBranchLib/Series RLC Branch  LConnTagsString=__new0  RConnTagsString=__new0  BranchType=RL  Resistance=0.6  Inductance=1e-6  SetiL0=off  InitialCurrent=0  Capacitance=1e-6  Setx0=off  InitialVoltage=0  Measurements=None
  Series RLC Branch9 : spsSeriesRLCBranchLib/Series RLC Branch  LConnTagsString=__new0  RConnTagsString=__new0  BranchType=L  Resistance=1  Inductance=0.4e-6  SetiL0=off  InitialCurrent=0  Capacitance=1e-6  Setx0=off  InitialVoltage=0  Measurements=None
  Terminator{,1..9} (10 alike) : Terminator
  Udc+ : PMIOPort  Side=Left
  udc- : PMIOPort  Port=2  Side=Left
  p1 : PMIOPort  Port=3  Side=Right
  p2 : PMIOPort  Port=4  Side=Right
  wires:
  Demux/4 -> [n1]
  Demux/2 -> [p1]
  Demux/1 -> [p2]
  PWM/1 -> Demux/1
  Demux/3 -> [n2]
  Diode6/1 -> Terminator1/1
  Diode1/1 -> Terminator6/1
  Diode8/1 -> Terminator7/1
  [p2] -> IGBT/1
  Diode2/1 -> Terminator8/1
  Current Measurement1/1 -> Terminator/1
  [p1] -> IGBT2/1
  [n2] -> IGBT1/1
  IGBT/1 -> Terminator2/1
  IGBT2/1 -> Terminator3/1
  IGBT1/1 -> Terminator4/1
  [n1] -> IGBT3/1
  IGBT3/1 -> Terminator5/1
  Diode3/1 -> Terminator9/1
  connections:
  IGBT/RConn1 -- Diode8/LConn1 -- Diode1/RConn1 -- IGBT1/LConn1 -- p2/RConn1
  Series RLC Branch9/RConn1 -- Series RLC Branch7/LConn1 -- Series RLC Branch1/LConn1
  Series RLC Branch2/RConn1 -- Series RLC Branch10/RConn1 -- Series RLC Branch14/LConn1 -- Series RLC Branch5/LConn1
  IGBT2/RConn1 -- IGBT3/LConn1 -- Diode3/RConn1 -- Diode2/LConn1 -- p1/RConn1
  IGBT2/LConn1 -- Series RLC Branch12/RConn1 -- Diode2/RConn1
  Current Measurement1/RConn1 -- Diode6/LConn1
  IGBT1/RConn1 -- Series RLC Branch5/RConn1 -- Diode1/LConn1
  Diode8/RConn1 -- IGBT/LConn1 -- Series RLC Branch3/RConn1
  Series RLC Branch14/RConn1 -- IGBT3/RConn1 -- Diode3/LConn1
  Series RLC Branch12/LConn1 -- Series RLC Branch3/LConn1 -- Series RLC Branch1/RConn1 -- Current Measurement1/LConn1
  Series RLC Branch2/LConn1 -- Series RLC Branch7/RConn1 -- Diode6/RConn1
  Series RLC Branch9/LConn1 -- Udc+/RConn1
  Series RLC Branch10/LConn1 -- udc-/RConn1

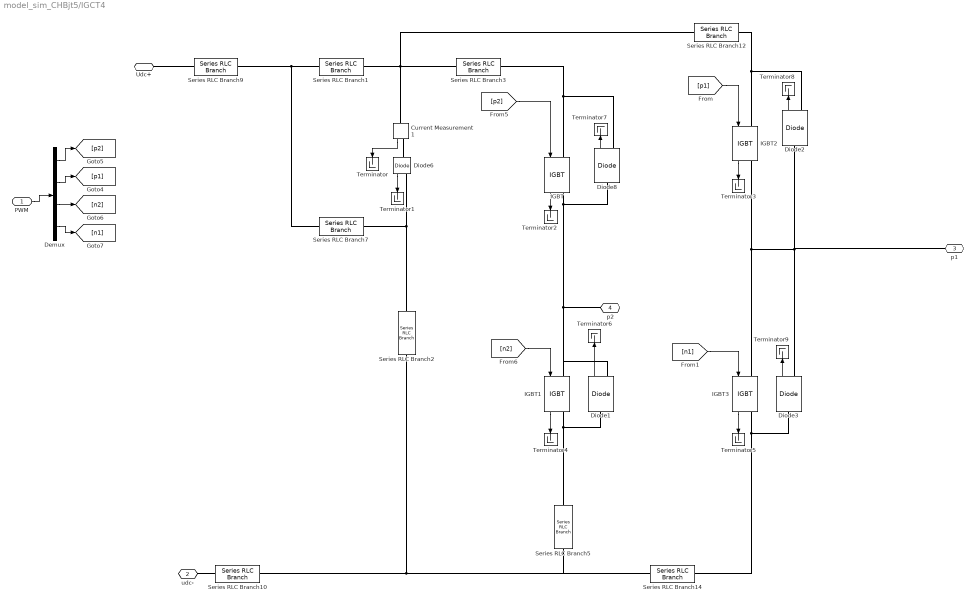
== system model_sim_CHBjt5/IGCT4 ==
  PWM : Inport
  Current Measurement1 : spsCurrentMeasurementLib/Current Measurement  PhasorSimulation=off  OutputType=Complex  PSBequivalent=0
  Demux : Demux
  Diode{1..3,6,8} (5 alike) : spsDiodeLib/Diode  Ron=rto  Lon=0  Vf=vto  IC=0  UseSnubber=off  Rs=500  Cs=250e-9  Measurements=on
  IGBT{,1..3} (4 alike) : spsIGBTLib/IGBT  Ron=rt  Lon=0  Vf=vt  Tf=1e-6  Tt=2e-6  IC=0  Rs=1e5  Cs=inf  Measurements=on
  Series RLC Branch1 : spsSeriesRLCBranchLib/Series RLC Branch  LConnTagsString=__new0  RConnTagsString=__new0  BranchType=RL  Resistance=1e-5  Inductance=3.0E-6  SetiL0=off  InitialCurrent=0  Capacitance=1e-6  Setx0=off  InitialVoltage=0  Measurements=None
  Series RLC Branch10 : spsSeriesRLCBranchLib/Series RLC Branch  LConnTagsString=__new0  RConnTagsString=__new0  BranchType=L  Resistance=1  Inductance=0.4e-6  SetiL0=off  InitialCurrent=0  Capacitance=1e-6  Setx0=off  InitialVoltage=0  Measurements=None
  Series RLC Branch12 : spsSeriesRLCBranchLib/Series RLC Branch  LConnTagsString=__new0  RConnTagsString=__new0  BranchType=RL  Resistance=1e-5  Inductance=1E-9  SetiL0=off  InitialCurrent=0  Capacitance=1e-6  Setx0=off  InitialVoltage=0  Measurements=None
  Series RLC Branch14 : spsSeriesRLCBranchLib/Series RLC Branch  LConnTagsString=__new0  RConnTagsString=__new0  BranchType=L  Resistance=1  Inductance=1E-7  SetiL0=off  InitialCurrent=0  Capacitance=1e-6  Setx0=off  InitialVoltage=0  Measurements=None
  Series RLC Branch2 : spsSeriesRLCBranchLib/Series RLC Branch  LConnTagsString=__new0  RConnTagsString=__new0  BranchType=RC  Resistance=1e-5  Inductance=20e-6  SetiL0=off  InitialCurrent=0  Capacitance=17e-6  Setx0=off  InitialVoltage=0  Measurements=None
  Series RLC Branch3 : spsSeriesRLCBranchLib/Series RLC Branch  LConnTagsString=__new0  RConnTagsString=__new0  BranchType=RL  Resistance=1e-5  Inductance=1E-9  SetiL0=off  InitialCurrent=0  Capacitance=1e-6  Setx0=off  InitialVoltage=0  Measurements=None
  Series RLC Branch5 : spsSeriesRLCBranchLib/Series RLC Branch  LConnTagsString=__new0  RConnTagsString=__new0  BranchType=L  Resistance=1  Inductance=1E-7  SetiL0=off  InitialCurrent=0  Capacitance=1e-6  Setx0=off  InitialVoltage=0  Measurements=None
  Series RLC Branch7 : spsSeriesRLCBranchLib/Series RLC Branch  LConnTagsString=__new0  RConnTagsString=__new0  BranchType=RL  Resistance=0.6  Inductance=1e-6  SetiL0=off  InitialCurrent=0  Capacitance=1e-6  Setx0=off  InitialVoltage=0  Measurements=None
  Series RLC Branch9 : spsSeriesRLCBranchLib/Series RLC Branch  LConnTagsString=__new0  RConnTagsString=__new0  BranchType=L  Resistance=1  Inductance=0.4e-6  SetiL0=off  InitialCurrent=0  Capacitance=1e-6  Setx0=off  InitialVoltage=0  Measurements=None
  Terminator{,1..9} (10 alike) : Terminator
  Udc+ : PMIOPort  Side=Left
  udc- : PMIOPort  Port=2  Side=Left
  p1 : PMIOPort  Port=3  Side=Right
  p2 : PMIOPort  Port=4  Side=Right
  wires:
  Demux/4 -> [n1]
  Demux/2 -> [p1]
  Demux/1 -> [p2]
  PWM/1 -> Demux/1
  Demux/3 -> [n2]
  Diode6/1 -> Terminator1/1
  Diode1/1 -> Terminator6/1
  Diode8/1 -> Terminator7/1
  [p2] -> IGBT/1
  Diode2/1 -> Terminator8/1
  Current Measurement1/1 -> Terminator/1
  [p1] -> IGBT2/1
  [n2] -> IGBT1/1
  IGBT/1 -> Terminator2/1
  IGBT2/1 -> Terminator3/1
  IGBT1/1 -> Terminator4/1
  [n1] -> IGBT3/1
  IGBT3/1 -> Terminator5/1
  Diode3/1 -> Terminator9/1
  connections:
  IGBT/RConn1 -- Diode8/LConn1 -- Diode1/RConn1 -- IGBT1/LConn1 -- p2/RConn1
  Series RLC Branch9/RConn1 -- Series RLC Branch7/LConn1 -- Series RLC Branch1/LConn1
  Series RLC Branch2/RConn1 -- Series RLC Branch10/RConn1 -- Series RLC Branch14/LConn1 -- Series RLC Branch5/LConn1
  IGBT2/RConn1 -- IGBT3/LConn1 -- Diode3/RConn1 -- Diode2/LConn1 -- p1/RConn1
  IGBT2/LConn1 -- Series RLC Branch12/RConn1 -- Diode2/RConn1
  Current Measurement1/RConn1 -- Diode6/LConn1
  IGBT1/RConn1 -- Series RLC Branch5/RConn1 -- Diode1/LConn1
  Diode8/RConn1 -- IGBT/LConn1 -- Series RLC Branch3/RConn1
  Series RLC Branch14/RConn1 -- IGBT3/RConn1 -- Diode3/LConn1
  Series RLC Branch12/LConn1 -- Series RLC Branch3/LConn1 -- Series RLC Branch1/RConn1 -- Current Measurement1/LConn1
  Series RLC Branch2/LConn1 -- Series RLC Branch7/RConn1 -- Diode6/RConn1
  Series RLC Branch9/LConn1 -- Udc+/RConn1
  Series RLC Branch10/LConn1 -- udc-/RConn1

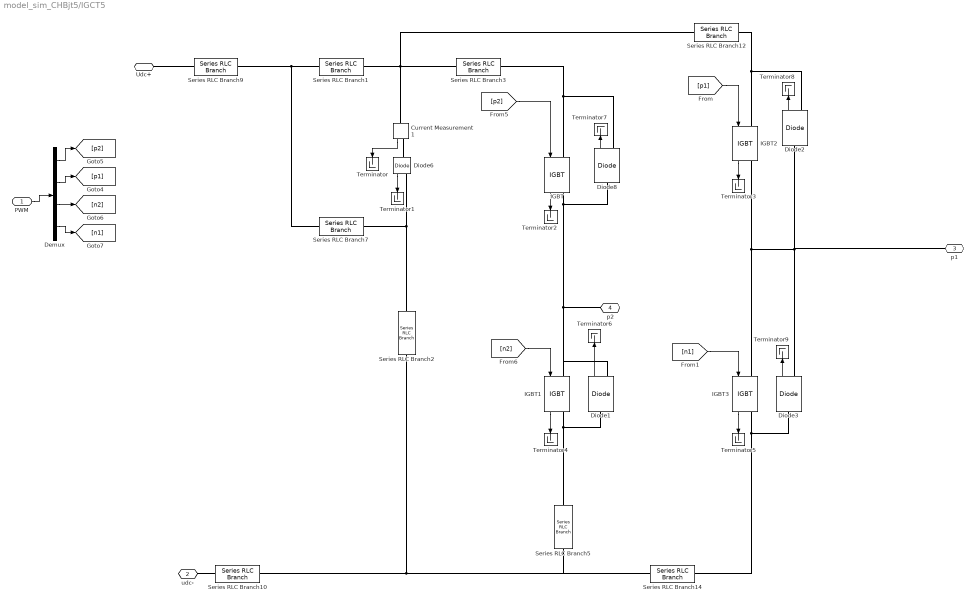
== system model_sim_CHBjt5/IGCT5 ==
  PWM : Inport
  Current Measurement1 : spsCurrentMeasurementLib/Current Measurement  PhasorSimulation=off  OutputType=Complex  PSBequivalent=0
  Demux : Demux
  Diode{1..3,6,8} (5 alike) : spsDiodeLib/Diode  Ron=rto  Lon=0  Vf=vto  IC=0  UseSnubber=off  Rs=500  Cs=250e-9  Measurements=on
  IGBT{,1..3} (4 alike) : spsIGBTLib/IGBT  Ron=rt  Lon=0  Vf=vt  Tf=1e-6  Tt=2e-6  IC=0  Rs=1e5  Cs=inf  Measurements=on
  Series RLC Branch1 : spsSeriesRLCBranchLib/Series RLC Branch  LConnTagsString=__new0  RConnTagsString=__new0  BranchType=RL  Resistance=1e-5  Inductance=3.0E-6  SetiL0=off  InitialCurrent=0  Capacitance=1e-6  Setx0=off  InitialVoltage=0  Measurements=None
  Series RLC Branch10 : spsSeriesRLCBranchLib/Series RLC Branch  LConnTagsString=__new0  RConnTagsString=__new0  BranchType=L  Resistance=1  Inductance=0.4e-6  SetiL0=off  InitialCurrent=0  Capacitance=1e-6  Setx0=off  InitialVoltage=0  Measurements=None
  Series RLC Branch12 : spsSeriesRLCBranchLib/Series RLC Branch  LConnTagsString=__new0  RConnTagsString=__new0  BranchType=RL  Resistance=1e-5  Inductance=1E-9  SetiL0=off  InitialCurrent=0  Capacitance=1e-6  Setx0=off  InitialVoltage=0  Measurements=None
  Series RLC Branch14 : spsSeriesRLCBranchLib/Series RLC Branch  LConnTagsString=__new0  RConnTagsString=__new0  BranchType=L  Resistance=1  Inductance=1E-7  SetiL0=off  InitialCurrent=0  Capacitance=1e-6  Setx0=off  InitialVoltage=0  Measurements=None
  Series RLC Branch2 : spsSeriesRLCBranchLib/Series RLC Branch  LConnTagsString=__new0  RConnTagsString=__new0  BranchType=RC  Resistance=1e-5  Inductance=20e-6  SetiL0=off  InitialCurrent=0  Capacitance=17e-6  Setx0=off  InitialVoltage=0  Measurements=None
  Series RLC Branch3 : spsSeriesRLCBranchLib/Series RLC Branch  LConnTagsString=__new0  RConnTagsString=__new0  BranchType=RL  Resistance=1e-5  Inductance=1E-9  SetiL0=off  InitialCurrent=0  Capacitance=1e-6  Setx0=off  InitialVoltage=0  Measurements=None
  Series RLC Branch5 : spsSeriesRLCBranchLib/Series RLC Branch  LConnTagsString=__new0  RConnTagsString=__new0  BranchType=L  Resistance=1  Inductance=1E-7  SetiL0=off  InitialCurrent=0  Capacitance=1e-6  Setx0=off  InitialVoltage=0  Measurements=None
  Series RLC Branch7 : spsSeriesRLCBranchLib/Series RLC Branch  LConnTagsString=__new0  RConnTagsString=__new0  BranchType=RL  Resistance=0.6  Inductance=1e-6  SetiL0=off  InitialCurrent=0  Capacitance=1e-6  Setx0=off  InitialVoltage=0  Measurements=None
  Series RLC Branch9 : spsSeriesRLCBranchLib/Series RLC Branch  LConnTagsString=__new0  RConnTagsString=__new0  BranchType=L  Resistance=1  Inductance=0.4e-6  SetiL0=off  InitialCurrent=0  Capacitance=1e-6  Setx0=off  InitialVoltage=0  Measurements=None
  Terminator{,1..9} (10 alike) : Terminator
  Udc+ : PMIOPort  Side=Left
  udc- : PMIOPort  Port=2  Side=Left
  p1 : PMIOPort  Port=3  Side=Right
  p2 : PMIOPort  Port=4  Side=Right
  wires:
  Demux/4 -> [n1]
  Demux/2 -> [p1]
  Demux/1 -> [p2]
  PWM/1 -> Demux/1
  Demux/3 -> [n2]
  Diode6/1 -> Terminator1/1
  Diode1/1 -> Terminator6/1
  Diode8/1 -> Terminator7/1
  [p2] -> IGBT/1
  Diode2/1 -> Terminator8/1
  Current Measurement1/1 -> Terminator/1
  [p1] -> IGBT2/1
  [n2] -> IGBT1/1
  IGBT/1 -> Terminator2/1
  IGBT2/1 -> Terminator3/1
  IGBT1/1 -> Terminator4/1
  [n1] -> IGBT3/1
  IGBT3/1 -> Terminator5/1
  Diode3/1 -> Terminator9/1
  connections:
  IGBT/RConn1 -- Diode8/LConn1 -- Diode1/RConn1 -- IGBT1/LConn1 -- p2/RConn1
  Series RLC Branch9/RConn1 -- Series RLC Branch7/LConn1 -- Series RLC Branch1/LConn1
  Series RLC Branch2/RConn1 -- Series RLC Branch10/RConn1 -- Series RLC Branch14/LConn1 -- Series RLC Branch5/LConn1
  IGBT2/RConn1 -- IGBT3/LConn1 -- Diode3/RConn1 -- Diode2/LConn1 -- p1/RConn1
  IGBT2/LConn1 -- Series RLC Branch12/RConn1 -- Diode2/RConn1
  Current Measurement1/RConn1 -- Diode6/LConn1
  IGBT1/RConn1 -- Series RLC Branch5/RConn1 -- Diode1/LConn1
  Diode8/RConn1 -- IGBT/LConn1 -- Series RLC Branch3/RConn1
  Series RLC Branch14/RConn1 -- IGBT3/RConn1 -- Diode3/LConn1
  Series RLC Branch12/LConn1 -- Series RLC Branch3/LConn1 -- Series RLC Branch1/RConn1 -- Current Measurement1/LConn1
  Series RLC Branch2/LConn1 -- Series RLC Branch7/RConn1 -- Diode6/RConn1
  Series RLC Branch9/LConn1 -- Udc+/RConn1
  Series RLC Branch10/LConn1 -- udc-/RConn1

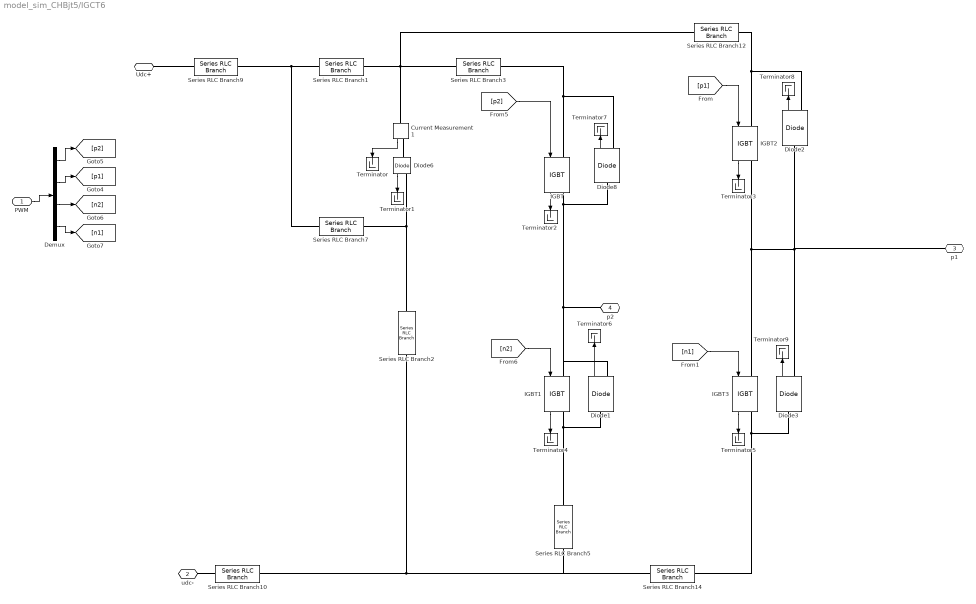
== system model_sim_CHBjt5/IGCT6 ==
  PWM : Inport
  Current Measurement1 : spsCurrentMeasurementLib/Current Measurement  PhasorSimulation=off  OutputType=Complex  PSBequivalent=0
  Demux : Demux
  Diode{1..3,6,8} (5 alike) : spsDiodeLib/Diode  Ron=rto  Lon=0  Vf=vto  IC=0  UseSnubber=off  Rs=500  Cs=250e-9  Measurements=on
  IGBT{,1..3} (4 alike) : spsIGBTLib/IGBT  Ron=rt  Lon=0  Vf=vt  Tf=1e-6  Tt=2e-6  IC=0  Rs=1e5  Cs=inf  Measurements=on
  Series RLC Branch1 : spsSeriesRLCBranchLib/Series RLC Branch  LConnTagsString=__new0  RConnTagsString=__new0  BranchType=RL  Resistance=1e-5  Inductance=3.0E-6  SetiL0=off  InitialCurrent=0  Capacitance=1e-6  Setx0=off  InitialVoltage=0  Measurements=None
  Series RLC Branch10 : spsSeriesRLCBranchLib/Series RLC Branch  LConnTagsString=__new0  RConnTagsString=__new0  BranchType=L  Resistance=1  Inductance=0.4e-6  SetiL0=off  InitialCurrent=0  Capacitance=1e-6  Setx0=off  InitialVoltage=0  Measurements=None
  Series RLC Branch12 : spsSeriesRLCBranchLib/Series RLC Branch  LConnTagsString=__new0  RConnTagsString=__new0  BranchType=RL  Resistance=1e-5  Inductance=1E-9  SetiL0=off  InitialCurrent=0  Capacitance=1e-6  Setx0=off  InitialVoltage=0  Measurements=None
  Series RLC Branch14 : spsSeriesRLCBranchLib/Series RLC Branch  LConnTagsString=__new0  RConnTagsString=__new0  BranchType=L  Resistance=1  Inductance=1E-7  SetiL0=off  InitialCurrent=0  Capacitance=1e-6  Setx0=off  InitialVoltage=0  Measurements=None
  Series RLC Branch2 : spsSeriesRLCBranchLib/Series RLC Branch  LConnTagsString=__new0  RConnTagsString=__new0  BranchType=RC  Resistance=1e-5  Inductance=20e-6  SetiL0=off  InitialCurrent=0  Capacitance=17e-6  Setx0=off  InitialVoltage=0  Measurements=None
  Series RLC Branch3 : spsSeriesRLCBranchLib/Series RLC Branch  LConnTagsString=__new0  RConnTagsString=__new0  BranchType=RL  Resistance=1e-5  Inductance=1E-9  SetiL0=off  InitialCurrent=0  Capacitance=1e-6  Setx0=off  InitialVoltage=0  Measurements=None
  Series RLC Branch5 : spsSeriesRLCBranchLib/Series RLC Branch  LConnTagsString=__new0  RConnTagsString=__new0  BranchType=L  Resistance=1  Inductance=1E-7  SetiL0=off  InitialCurrent=0  Capacitance=1e-6  Setx0=off  InitialVoltage=0  Measurements=None
  Series RLC Branch7 : spsSeriesRLCBranchLib/Series RLC Branch  LConnTagsString=__new0  RConnTagsString=__new0  BranchType=RL  Resistance=0.6  Inductance=1e-6  SetiL0=off  InitialCurrent=0  Capacitance=1e-6  Setx0=off  InitialVoltage=0  Measurements=None
  Series RLC Branch9 : spsSeriesRLCBranchLib/Series RLC Branch  LConnTagsString=__new0  RConnTagsString=__new0  BranchType=L  Resistance=1  Inductance=0.4e-6  SetiL0=off  InitialCurrent=0  Capacitance=1e-6  Setx0=off  InitialVoltage=0  Measurements=None
  Terminator{,1..9} (10 alike) : Terminator
  Udc+ : PMIOPort  Side=Left
  udc- : PMIOPort  Port=2  Side=Left
  p1 : PMIOPort  Port=3  Side=Right
  p2 : PMIOPort  Port=4  Side=Right
  wires:
  Demux/4 -> [n1]
  Demux/2 -> [p1]
  Demux/1 -> [p2]
  PWM/1 -> Demux/1
  Demux/3 -> [n2]
  Diode6/1 -> Terminator1/1
  Diode1/1 -> Terminator6/1
  Diode8/1 -> Terminator7/1
  [p2] -> IGBT/1
  Diode2/1 -> Terminator8/1
  Current Measurement1/1 -> Terminator/1
  [p1] -> IGBT2/1
  [n2] -> IGBT1/1
  IGBT/1 -> Terminator2/1
  IGBT2/1 -> Terminator3/1
  IGBT1/1 -> Terminator4/1
  [n1] -> IGBT3/1
  IGBT3/1 -> Terminator5/1
  Diode3/1 -> Terminator9/1
  connections:
  IGBT/RConn1 -- Diode8/LConn1 -- Diode1/RConn1 -- IGBT1/LConn1 -- p2/RConn1
  Series RLC Branch9/RConn1 -- Series RLC Branch7/LConn1 -- Series RLC Branch1/LConn1
  Series RLC Branch2/RConn1 -- Series RLC Branch10/RConn1 -- Series RLC Branch14/LConn1 -- Series RLC Branch5/LConn1
  IGBT2/RConn1 -- IGBT3/LConn1 -- Diode3/RConn1 -- Diode2/LConn1 -- p1/RConn1
  IGBT2/LConn1 -- Series RLC Branch12/RConn1 -- Diode2/RConn1
  Current Measurement1/RConn1 -- Diode6/LConn1
  IGBT1/RConn1 -- Series RLC Branch5/RConn1 -- Diode1/LConn1
  Diode8/RConn1 -- IGBT/LConn1 -- Series RLC Branch3/RConn1
  Series RLC Branch14/RConn1 -- IGBT3/RConn1 -- Diode3/LConn1
  Series RLC Branch12/LConn1 -- Series RLC Branch3/LConn1 -- Series RLC Branch1/RConn1 -- Current Measurement1/LConn1
  Series RLC Branch2/LConn1 -- Series RLC Branch7/RConn1 -- Diode6/RConn1
  Series RLC Branch9/LConn1 -- Udc+/RConn1
  Series RLC Branch10/LConn1 -- udc-/RConn1
